simulink model "Assignment1_final_bonus_take1000"  (R2017b)
settings: Solver=FixedStepAuto  StartTime=0.0  StopTime=inf  FixedStep=0.001  RelTol=1e-3  EnableMultiTasking=on
undefined symbols (not defined in the file): D10, D11, D12, D2, D5, D8, D9, PTA0, PTA2, PTB9, PTC4, PTD0, PTD2, PTD3
libraries: frdmk64flib x10
settings Model: ExtModeTrigDuration=5  Creator=montema2  LastModifiedBy=brydoa1
settings OptimizationCC: PassReuseOutputArgsAs=Individual arguments  MaxStackSize=64
settings DebuggingCC: ParameterTunabilityLossMsg=error
settings HardwareCC: ProdBitPerPointer=32  ProdBitPerSizeT=32  ProdBitPerPtrDiffT=32  ProdLargestAtomicInteger=Long  ProdLargestAtomicFloat=Double  ProdWordSize=32  ProdHWDeviceType=ARM Compatible->ARM Cortex
settings SFSimCC: MATLABDynamicMemAlloc=off
settings RTWCC: SystemTargetFile=ert.tlc  HardwareBoard=NXP FRDM-K64F  TemplateMakefile=ert_default_tmf  GenerateReport=on  Toolchain=GNU Tools for ARM Embedded Processors  IncludeHyperlinkInReport=on  LaunchReport=on  GenerateTraceInfo=on  GenerateTraceReport=on  GenerateTraceReportSl=on  GenerateTraceReportSf=on  GenerateTraceReportEml=on
settings CodeAppCC: ForceParamTrailComments=on  IgnoreCustomStorageClasses=off  OperatorAnnotations=on  SimulinkDataObjDesc=on  SFDataObjDesc=on  InsertBlockDesc=on

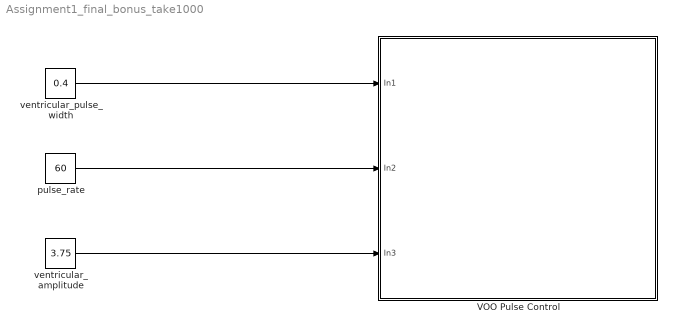
== system Assignment1_final_bonus_take1000 ==
  VOO Pulse Control : Subsystem
  pulse_rate : Constant  Value=60
  ventricular_amplitude : Constant  Value=3.75
  ventricular_pulse_width : Constant  Value=0.4
  wires:
  ventricular_pulse_width/1 -> VOO Pulse Control/1(In1)
  pulse_rate/1 -> VOO Pulse Control/2(In2)
  ventricular_amplitude/1 -> VOO Pulse Control/3(In3)

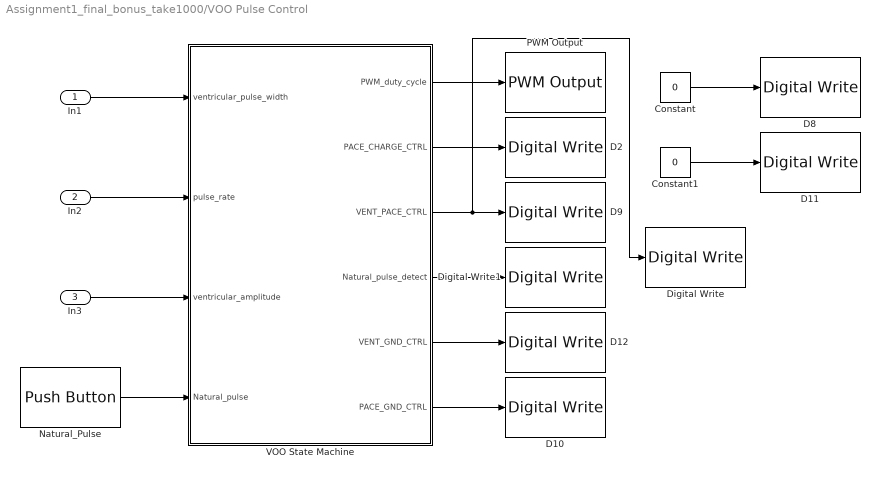
== system Assignment1_final_bonus_take1000/VOO Pulse Control ==
  In1 : Inport
  In2 : Inport  Port=2
  In3 : Inport  Port=3
  Constant : Constant  Value=0
  Constant1 : Constant  Value=0
  D10 : frdmk64flib/Digital Write  Whichpin=PTD0 (D10)
      settings: SourceProductName=Simulink Coder Support Package for NXP FRDM-K64F Board
  D11 : frdmk64flib/Digital Write  Whichpin=PTD2 (D11)
      settings: SourceProductName=Simulink Coder Support Package for NXP FRDM-K64F Board
  D12 : frdmk64flib/Digital Write  Whichpin=PTD3 (D12)
      settings: SourceProductName=Simulink Coder Support Package for NXP FRDM-K64F Board
  D2 : frdmk64flib/Digital Write  Whichpin=PTB9 (D2)
      settings: SourceProductName=Simulink Coder Support Package for NXP FRDM-K64F Board
  D8 : frdmk64flib/Digital Write  Whichpin=PTA0 (D8)
      settings: SourceProductName=Simulink Coder Support Package for NXP FRDM-K64F Board
  D9 : frdmk64flib/Digital Write  Whichpin=PTC4 (D9)
      settings: SourceProductName=Simulink Coder Support Package for NXP FRDM-K64F Board
  Digital Write : frdmk64flib/Digital Write  Whichpin=RED_LED
      settings: SourceProductName=Simulink Coder Support Package for NXP FRDM-K64F Board
  Digital Write1 : frdmk64flib/Digital Write  Whichpin=BLUE_LED
      settings: SourceProductName=Simulink Coder Support Package for NXP FRDM-K64F Board
  Natural_Pulse : frdmk64flib/Push Button  Whichswitch=SW2  SampleTime1=-1
      settings: SourceProductName=Simulink Coder Support Package for NXP FRDM-K64F Board
  PWM Output : frdmk64flib/PWM Output  Whichpin=PTA2 (D5)  InitialFrequency=1000  InitialDutyCycle=0
      settings: SourceProductName=Simulink Coder Support Package for NXP FRDM-K64F Board
  VOO State Machine : Stateflow chart  TreatAsAtomicUnit=on
  wires:
  In1/1 -> VOO State Machine/1(ventricular_pulse_width)
  VOO State Machine/1(PWM_duty_cycle) -> PWM Output/1
  VOO State Machine/3(VENT_PACE_CTRL) -> Digital Write/1, D9/1
  In2/1 -> VOO State Machine/2(pulse_rate)
  VOO State Machine/2(PACE_CHARGE_CTRL) -> D2/1
  VOO State Machine/5(VENT_GND_CTRL) -> D12/1
  VOO State Machine/6(PACE_GND_CTRL) -> D10/1
  Constant/1 -> D8/1
  Constant1/1 -> D11/1
  Natural_Pulse/1 -> VOO State Machine/4(Natural_pulse)
  VOO State Machine/4(Natural_pulse_detect) -> Digital Write1/1
  In3/1 -> VOO State Machine/3(ventricular_amplitude)

== stateflow chart Assignment1_final_bonus_take1000/VOO Pulse Control/VOO State Machine ==
  note: Switch States:
      | true=closed
      | false=open
  state start_state
    entry:VENT_PACE_CTRL=false;
    VENT_GND_CTRL=true;
    PACE_CHARGE_CTRL=true;
    PACE_GND_CTRL=true;
    PWM_duty_cycle=((ventricular_amplitude/5)*100);
  state current_into_heart
    entry:
    PACE_CHARGE_CTRL=false;
    VENT_GND_CTRL=false;
    VENT_PACE_CTRL=true;
  state current_out_of_heart
    entry:
    VENT_PACE_CTRL=false;
    PACE_CHARGE_CTRL=true;
    VENT_GND_CTRL=true;
  state natural_pace
    entry: Natural_pulse_detect=true;
    exit: Natural_pulse_detect=false;
  (default) -> start_state
  start_state -> current_into_heart [order 1] : [after(((60/pulse_rate)*1000),msec)]
  current_into_heart -> natural_pace [order 2] : [Natural_pulse==true]
  start_state -> natural_pace [order 2] : [Natural_pulse==true]
  natural_pace -> start_state : [Natural_pulse==false]
  current_into_heart -> current_out_of_heart [order 1] : [after((ventricular_pulse_width),msec)]
  current_out_of_heart -> current_into_heart [order 1] : [after(((60/pulse_rate)*1000)-(ventricular_pulse_width),msec)]
  current_out_of_heart -> natural_pace [order 2] : [Natural_pulse==true]
  data: ventricular_pulse_width input double; pulse_rate input double; ventricular_amplitude input double; PWM_duty_cycle output double [0..100]; PACE_CHARGE_CTRL output boolean; VENT_PACE_CTRL output boolean; Natural_pulse_detect output; VENT_GND_CTRL output boolean; PACE_GND_CTRL output boolean; Natural_pulse input boolean
